simulink model "ardupilotsailboat"  (R2024a)
settings: Solver=ode15s  StartTime=0.0  StopTime=2  RelTol=1e-3
values from neighbouring files (symbols this model uses):
  Ixx = 1/120 * pi * rho * L * B * T * (4*T^2 + B^2)    (= 0.835683076278)    [parameterCalculations.m]
  Izz = 1/120 * pi * rho * L * B * T * (B^2 + L^2)    (= 1.17027496573)    [parameterCalculations.m]
  m = 2.7    [parameterCalculations.m]
  m11 = m*k11    [parameterCalculations.m]
  m22 = m*k22    [parameterCalculations.m]
  m24 = 0    [parameterCalculations.m]
  m26 = xb*m22    [parameterCalculations.m]
  m66 = k66*Izz    [parameterCalculations.m]
  Nr = -pi * T^2/L^2 * (0.25 +0.039 * B/T - 0.56 * B/L)    (= -0.104988463049)    [parameterCalculations.m]
  Nv = -pi * T^2/L^2 * (0.5 +2.4 * T/L)    (= -0.841300100031)    [parameterCalculations.m]
  Yv = -pi * T^2/L^2 * (1 +0.4 * CB * B/T)    (= -0.560439243466)    [parameterCalculations.m]
undefined symbols (not defined in the file or in its folder): Waypoints
libraries: cstblocks x6, simulink x4, vrlib x1
(part 1 of 2)
settings Model: Creator=ruben  LastModifiedBy=ruben
settings SolverCC: MaxConsecutiveZCs=10  MaxConsecutiveMinStep=12  ZeroCrossControl=EnableAll  ZeroCrossAlgorithm=Adaptive  SolverResetMethod=Robust  DecoupledContinuousIntegration=on
settings OptimizationCC: ReuseModelBlockBuffer=off
settings DebuggingCC: SignalInfNanChecking=warning  AlgebraicLoopMsg=error  ArtificialAlgebraicLoopMsg=error  BlockPriorityViolationMsg=error  MinStepSizeMsg=error  MaskedZcDiagnostic=error  IgnoredZcDiagnostic=none  MultiTaskCondExecSysMsg=warning  MultiTaskRateTransMsg=warning  CheckMatrixSingularityMsg=error  StateNameClashWarn=warning
settings RTWCC: GPUComputeCapability=3.5

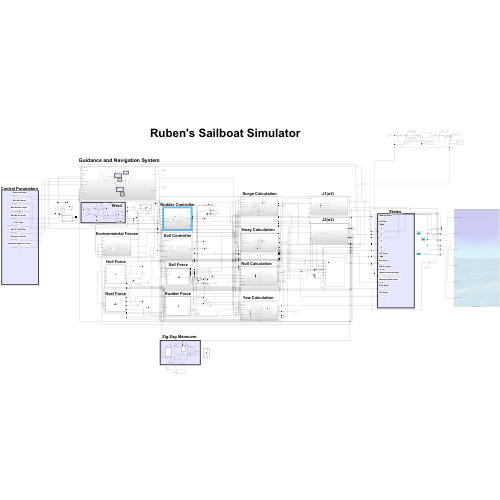
[thumbnail: Simulink's stored preview of the top-level diagram]
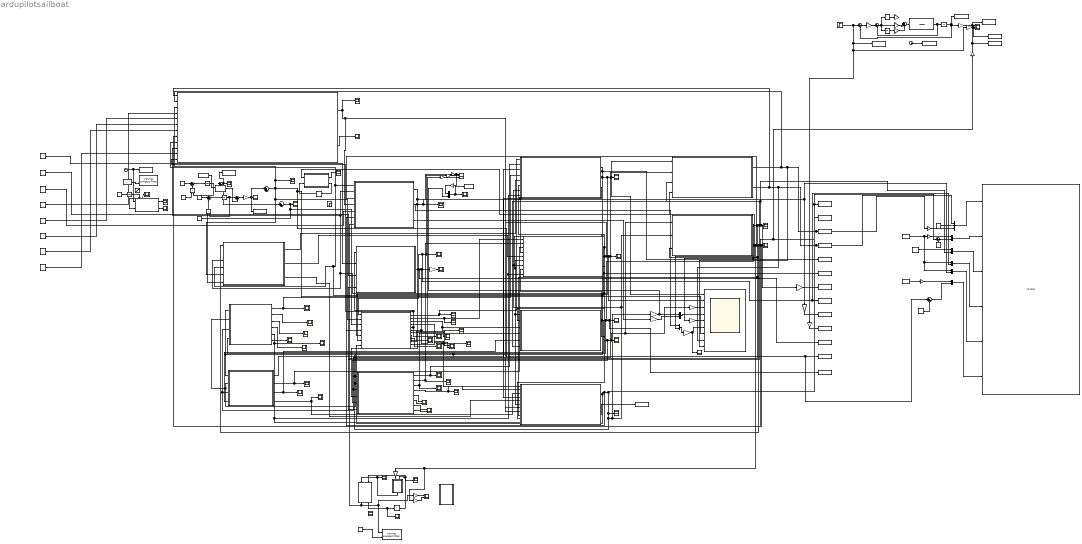
== system ardupilotsailboat ==
  note: Sail Force
  note: Ruben's Sailboat Simulator
  note: States
  note: x
  note: y
  note: Yaw Rate
  note: Heading Angle
  note: u
  note: v
  note: Roll Angle
  note: Sail Angle
  note: Rudder Angle
  note: Desired Heading Angle
  note: Apparent Wind Angle
  note: Wind Angle
  note: Roll Angle
  note: Guidance and Navigation System
  note: Environmental Forces
  note: Surge Calculation
  note: Sway Calculation
  note: Roll Calculation
  note: Yaw Calculation
  note: Wind
  note: Rudder Force
  note: Keel Force
  note: Hull Force
  note: Sail Controller
  note: Rudder Controller
  note: Zig-Zag Maneuver
  note: Control Parameters
  note: Max Sail Angle
  note: Min Sail Angle
  note: Sail No Go Angle
  note: Sail X-Track Max
  note: Waypoint Approach Side
  note: Waypoint Radius
  note: Tack Type
  note: Max Rudder Angle
  note: J1(n2)
  note: J2(n2)
  Band-Limited White Noise : simulink/Sources/Band-Limited White Noise  Cov=[0.05]  Ts=0.25  seed=[23341]
  Band-Limited White Noise1 : simulink/Sources/Band-Limited White Noise  Cov=[0.2]  Ts=0.01  seed=[3341]
  Band-Limited White Noise2 : simulink/Sources/Band-Limited White Noise  Cov=[0.4]  Ts=0.01  seed=[23341]
  Bus Creator : BusCreator  Inputs=2
  Bus Creator1 : BusCreator  Inputs=2
  Bus Creator2 : BusCreator  Inputs=2
  Clock : Clock
  Clock2 : Clock
  Constant : Constant  Value=0.5
  Constant1 : Constant  Value=1.56
  Constant2 : Constant  Value=0.5
  Constant3 : Constant  Value=0
  Cross-Track Distance(m) : Constant  Value=10
  Delay1 : Delay  DelayLength=1  SampleTime=0.01
  Delay2 : Delay  DelayLength=1  SampleTime=0.01
  Derivative : Derivative
  Gain : Gain  Gain=0.0225
  Gain{1..7,12..19,21..22} (17 alike) : Gain  Gain=180/pi
  Gain10 : Gain  Gain=0.332
  Gain11 : Gain
  Gain20 : Gain
  Gain23 : Gain
  Gain8 : Gain  Gain=-180/pi
  Gain9 : Gain  Gain=0.667
  Integrator{,1..2,4} (4 alike) : Integrator
  Integrator3 : Integrator  UpperSaturationLimit=1.3  LowerSaturationLimit=-1.3
  MATLAB Function1 : MATLAB Function  TreatAsAtomicUnit=on
  MATLAB Function2 : MATLAB Function  TreatAsAtomicUnit=on
  MATLAB Function3 : MATLAB Function  TreatAsAtomicUnit=on
  MATLAB Function4 : MATLAB Function  TreatAsAtomicUnit=on
  MATLAB Function5 : MATLAB Function  TreatAsAtomicUnit=on
  MATLAB Function6 : MATLAB Function  TreatAsAtomicUnit=on
  MATLAB Function7 : MATLAB Function  TreatAsAtomicUnit=on
  MATLAB Function8 : MATLAB Function  TreatAsAtomicUnit=on
  MATLAB Function9 : MATLAB Function  TreatAsAtomicUnit=on
  Mux1 : Mux  Inputs=3
  Mux{2,4..7} (5 alike) : Mux  Inputs=2
  "Port: 0, Starboard:1" : Constant  Value=0
  Product : Product
  Product1 : Product
  Radius of Acceptance(m) : Constant  Value=5
  Roll Axis of Rotation : Constant  Value=[ 1 0 0 ]
  Saturation1 : Saturate  UpperLimit=pi/18  LowerLimit=-pi/18
  Scope{,1..14,16..17,19..30,33..35,37..40,42..44} (39 alike) : Scope
  Scope15 : Scope  NumInputPorts=3
  Scope18 : Scope  NumInputPorts=3
  Scope31 : Scope  NumInputPorts=2
  Scope32 : Scope  NumInputPorts=2
  Scope36 : Scope  NumInputPorts=9
  Scope41 : Scope  NumInputPorts=2
  Step : Step  After=0  SampleTime=0
  Step2 : Step  After=0.25  SampleTime=0
  Subsystem1 : Subsystem
  Subsystem10 : Subsystem
  Subsystem2 : Subsystem
  Subsystem3 : Subsystem
  Subsystem4 : Subsystem
  Subsystem5 : Subsystem
  Subsystem6 : Subsystem
  Subsystem7 : Subsystem
  Subsystem8 : Subsystem
  Subsystem9 : Subsystem
  Sum{,5,8,10} (4 alike) : Sum  Inputs=|++
  Sum1 : Sum  Inputs=|+-  SaturateOnIntegerOverflow=on
  Sum{2,4,6..7,9} (5 alike) : Sum  Inputs=|+-
  Sum3 : Sum  Inputs=|+++
  "Tack Type (1:Direct, 2:Indirect 3:Zone)" : Constant
  To File : ToFile  Filename=sim_step.mat  SaveFormat=Timeseries
  To Workspace : ToWorkspace  VariableName=yawrate  SaveFormat=Timeseries  SampleTime=-1
  To Workspace1 : ToWorkspace  VariableName=yaw  SaveFormat=Timeseries  SampleTime=-1
  To Workspace10 : ToWorkspace  VariableName=psid  SaveFormat=Timeseries  SampleTime=-1
  To Workspace11 : ToWorkspace  VariableName=awa  SaveFormat=Timeseries  SampleTime=-1
  To Workspace12 : ToWorkspace  VariableName=wind  SaveFormat=Timeseries  SampleTime=-1
  To Workspace13 : ToWorkspace  VariableName=roll  SaveFormat=Timeseries  SampleTime=-1
  To Workspace14 : ToWorkspace  VariableName=time1  SaveFormat=Timeseries  SampleTime=-1
  To Workspace15 : ToWorkspace  VariableName=time  SaveFormat=Timeseries  SampleTime=-1
  To Workspace16 : ToWorkspace  VariableName=step  SaveFormat=Timeseries  SampleTime=-1
  To Workspace17 : ToWorkspace  VariableName=firstOrder  SaveFormat=Timeseries  SampleTime=-1
  To Workspace18 : ToWorkspace  VariableName=stepInput  SaveFormat=Timeseries  SampleTime=-1
  To Workspace19 : ToWorkspace  VariableName=nonLinear  SaveFormat=Timeseries  SampleTime=-1
  To Workspace2 : ToWorkspace  VariableName=simout  SaveFormat=Timeseries  SampleTime=-1
  To Workspace20 : ToWorkspace  VariableName=yawaccel  SaveFormat=Timeseries  SampleTime=-1
  To Workspace21 : ToWorkspace  VariableName=speed  SaveFormat=Timeseries  SampleTime=-1
  To Workspace22 : ToWorkspace  VariableName=direction  SaveFormat=Timeseries  SampleTime=-1
  To Workspace3 : ToWorkspace  VariableName=x  SaveFormat=Timeseries  SampleTime=-1
  To Workspace4 : ToWorkspace  VariableName=y  SaveFormat=Timeseries  SampleTime=-1
  To Workspace5 : ToWorkspace  VariableName=u  SaveFormat=Timeseries  SampleTime=-1
  To Workspace6 : ToWorkspace  VariableName=v  SaveFormat=Timeseries  SampleTime=-1
  To Workspace7 : ToWorkspace  VariableName=phi  SaveFormat=Timeseries  SampleTime=-1
  To Workspace8 : ToWorkspace  VariableName=delta_s  SaveFormat=Timeseries  SampleTime=-1
  To Workspace9 : ToWorkspace  VariableName=delta_r  SaveFormat=Timeseries  SampleTime=-1
  Transfer Fcn : TransferFcn  Numerator=[2.1]  Denominator=[0.1 1 ]
  VR Sailing Yacht Animation : vrlib/VR Sink  InstantiateOnLoad=on  SampleTime=0.05  ViewEnable=on  RemoteChange=off  RemoteView=off  FieldsWritten=Hull_EarthFixed.translation.3.1.1.double#Rot_Yaw.rotation.4.1.1.double#Rot_Roll.rotation.4.1.1.double#Sail.rotation.4.1.1.double#Rudder.rotation.4.1.1.double#Wind_Arrow.rotation.4.1.1.double  WorldFileName=SailingYachtAnimation.wrl  WorldDescription=Sailing Yacht VR animation  AutoView=on  VideoDimensions=[]  AllowVariableSize=off  FigureProperties="{'Position', 'Name', 'Viewpoint', 'CameraBound', 'CameraDirection', 'CameraPosition', 'CameraUpVector', 'ZoomFactor', 'Antialiasing', 'Headlight', 'Lighting', 'Sound', 'StatusBar', 'Stereo3D', 'Stereo3DCameraOffset', 'Stereo3DHIT', 'ToolBar', 'Textures', 'Transparency', 'Triad', 'Wireframe', 'NavZones', 'NavMode', 'NavSpeed', 'CaptureFileFormat', 'CaptureFileName', 'Record2DCompressMethod', 'Record2DCompressQuality', 'Record2D', 'Record2DFileName', 'Record2DFPS', 'NavPanel'; [-1.9180000000000000e+03   1.6800000000000000e+02   9.5800000000000000e+02   3.8000000000000000e+02], 'Sailing Yacht VR animation', 'Stern', 'on', [4.7333818472333400e-01  -2.7328284422274179e-01  -8.3741713019040154e-01], [-6.4413875659303592e+00   1.1181180118629433e+01   1.9816976942940634e+01], [9.7174256959609767e-02   9.6105616995744136e-01  -2.5870485494298978e-01], [1.0000000000000000e+00], 'on', 'on', 'on', 'on', 'on', 'off', [1.0000000149011612e-01], [0.0000000000000000e+00], 'on', 'on', 'on', 'none', 'off', 'off', 'fly', 'normal', 'tif', '%f_anim_%n.tif', 'auto', [7.5000000000000000e+01], 'off', '%f_anim_%n.avi', 'auto', 'halfbar'}"
  Varying Lowpass Filter : cstblocks/Linear Parameter Varying/Varying Lowpass Filter  N=1
  Varying Lowpass Filter1 : cstblocks/Linear Parameter Varying/Varying Lowpass Filter  N=1
  Yaw Axis of Rotation : Constant  Value=[ 0 1 0 ]
  Yaw Axis of Rotation1 : Constant  Value=[ 0 1 0 ]
  apparent wind : Scope
  fr2 : Constant  Value=20
  freq : Constant  Value=2
  max rudder angle(Rad) : Constant  Value=pi/6
  max sail angle(Rad) : Constant  Value=pi/3
  min sail angle(Rad) : Constant  Value=-pi/3
  pi : Constant  Value=pi
  rudder and psi1 : Scope  NumInputPorts=2
  rudder angle{1,5..6,8} (4 alike) : Scope
  rudder_angle1 : Scope
  rudder_angle2 : Scope
  sail angle : Scope
  sail no go angle(Degrees) : Constant  Value=60
  z : Constant  Value=0
  z - y1 : Gain
  z - y2 : Gain  Gain=-1
  z - y3 : Gain
  z1 : Constant  Value=pi/2
  wires:
  Subsystem1/2(heading (degrees)) -> Scope33/1
  MATLAB Function3/2(Ys) -> Scope1/1, Subsystem4/1(sail force (Ys))
  MATLAB Function3/3(Ks) -> Scope14/1, Subsystem5/3(sail force (Ks))
  MATLAB Function3/4(Ns) -> Subsystem6/1(sail force (Ns)), Scope23/1
  MATLAB Function4/2(Yr) -> Scope2/1, Subsystem4/2(rudder force (Yr))
  MATLAB Function4/3(Kr) -> Scope13/1, Subsystem5/4(roll angle)
  MATLAB Function5/1(Xk) -> Subsystem2/3(keel force (Xk))
  MATLAB Function5/2(Yk) -> Scope3/1, Subsystem4/3(keel force (Yk))
  MATLAB Function5/3(Kk) -> Scope12/1, Subsystem5/5(keel force (Kk))
  MATLAB Function5/4(Nk) -> Scope25/1, Subsystem6/3(keel force (Nk))
  MATLAB Function6/1(Xh) -> Scope5/1, Subsystem2/4(hull force (Xh))
  MATLAB Function6/3(Kh) -> Scope11/1
  MATLAB Function6/4(Nh) -> Scope24/1
  Subsystem4/1(v) -> To Workspace6/1, MATLAB Function3/6(v), Subsystem2/6(v), Subsystem6/7(v), Scope36/2, Scope8/1, Subsystem9/2(v), MATLAB Function6/3(v), MATLAB Function5/3(v), MATLAB Function4/3(v), Subsystem5/2(v), Subsystem8/2(v), Subsystem1/10(v), Subsystem3/3(v)
  Subsystem3/1(Xe) -> Subsystem2/5(environmental force (Xe))
  Subsystem3/2(Ye) -> Subsystem4/5(environmental force (Ye))
  Subsystem3/3(Ne) -> Subsystem6/5(environmental force (Ne))
  Subsystem2/1(u) -> MATLAB Function5/2(u), MATLAB Function6/2(u), MATLAB Function4/2(u), Subsystem1/9(u), Subsystem8/1(u), Subsystem3/4(u), Subsystem6/6(u), Subsystem5/1(u), Subsystem4/6(u), MATLAB Function3/5(u), Scope36/1, Subsystem9/1(u), Scope35/1, To Workspace5/1
  Subsystem5/1(p) -> MATLAB Function4/5(p), Subsystem10/1(p), Gain5/1, Scope38/1, Subsystem4/8(p)
  Subsystem10/1(Phi) -> Gain3/1, MATLAB Function5/4(phi), MATLAB Function6/4(phi), To Workspace13/1, Scope37/1, Subsystem6/9(roll), Subsystem7/4(roll_angle), Subsystem10/3(phi), MATLAB Function4/6(phi), Subsystem9/3(phi), Gain22/1, Scope9/1, Subsystem5/6(rudder force (Kr)), Mux6/2
  Clock2/1 -> MATLAB Function2/1(t), To Workspace14/1
  MATLAB Function7/2(nextState) -> rudder angle5/1, Delay1/1
  Delay1/1 -> rudder angle8/1, MATLAB Function8/2(state), MATLAB Function7/2(currentState)
  MATLAB Function8/1(y) -> MATLAB Function7/1(r), rudder angle1/1
  Gain2/1 -> rudder and psi1/1
  Subsystem7/1(sail angle) -> Gain7/1, sail angle/1, Mux5/2, To Workspace8/1, MATLAB Function3/1(delta_s)
  MATLAB Function3/6(alpha_aw) -> Gain6/1, To Workspace11/1, Gain14/1
  Subsystem8/1(rudder angle) -> Gain8/1, Gain18/1, Mux7/2, rudder_angle1/1, MATLAB Function4/4("delta_r ")
  MATLAB Function4/5(delta_r) -> Scope41/1
  MATLAB Function4/6(alpha_a) -> Scope41/2
  max sail angle(Rad)/1 -> Subsystem7/2(max sail angle)
  min sail angle(Rad)/1 -> Subsystem7/3(min sail angle)
  max rudder angle(Rad)/1 -> Subsystem8/5(max rudder angle)
  sail no go angle(Degrees)/1 -> Subsystem1/4(no go Angle)
  "Tack Type (1:Direct, 2:Indirect 3:Zone)"/1 -> Subsystem1/5(tack Type)
  Cross-Track Distance(m)/1 -> Subsystem1/6(Cross-Track Distance)
  Radius of Acceptance(m)/1 -> Subsystem1/7(radius of acceptance)
  Gain23/1 -> Sum/1, To Workspace22/1, Scope43/1
  MATLAB Function6/5(Frh) -> Scope6/1
  MATLAB Function3/1(Xs) -> Subsystem2/1(sail force (Xs)), Scope7/1
  Subsystem9/2(y) -> Subsystem1/1(x position of Sailboat), Scope36/8, Mux1/1, To Workspace3/1
  Subsystem8/2(Desired Heading) -> Bus Creator/1
  Subsystem10/2(Psi) -> MATLAB Function1/1(psi), Bus Creator/2, Subsystem9/4(psi), Gain17/1, Sum1/1, To Workspace1/1, Subsystem1/8(psi), MATLAB Function3/4(psi), Scope10/1, Subsystem3/1(psi), Subsystem8/3(psi), Gain12/1, Gain13/1
  Bus Creator/1 -> Gain1/1
  z1/1 -> Sum1/2
  z - y1/1 -> Mux4/1
  Yaw Axis of Rotation/1 -> Mux5/1, Mux7/1, z - y1/1
  z/1 -> Mux1/2
  z - y3/1 -> Mux2/1
  Mux2/1 -> VR Sailing Yacht Animation/6
  Sum1/1 -> Mux4/2
  Yaw Axis of Rotation1/1 -> z - y3/1
  z - y2/1 -> Mux1/3
  Roll Axis of Rotation/1 -> Mux6/1
  Mux1/1 -> VR Sailing Yacht Animation/1
  Mux4/1 -> VR Sailing Yacht Animation/2
  Mux6/1 -> VR Sailing Yacht Animation/3
  Mux5/1 -> VR Sailing Yacht Animation/4
  Mux7/1 -> VR Sailing Yacht Animation/5
  Subsystem9/1(x) -> Subsystem1/2(y position of Sailboat), Scope36/9, z - y2/1, To Workspace4/1
  MATLAB Function3/5(awa) -> Subsystem7/1(apparent_wind_angle), Subsystem1/12(awa), Scope42/1
  Gain3/1 -> Scope36/5
  Gain1/1 -> Scope19/1, Scope36/6
  Gain4/1 -> Bus Creator2/1, Bus Creator1/2
  Gain5/1 -> Scope36/3
  Gain6/1 -> Scope15/3
  Gain7/1 -> Scope15/2
  Gain8/1 -> Gain20/1, Scope15/1
  MATLAB Function1/2(nextState) -> Delay2/1
  Delay2/1 -> MATLAB Function1/2(currentState)
  MATLAB Function1/1(y) -> Scope16/1
  Clock/1 -> To Workspace15/1
  Integrator/1 -> Gain10/1
  Derivative/1 -> Gain/1
  Gain9/1 -> Sum3/2
  Transfer Fcn/1 -> Sum2/2, Integrator1/1
  Sum2/1 -> Derivative/1, Gain9/1, Integrator/1
  Sum3/1 -> Transfer Fcn/1
  Gain10/1 -> Sum3/3
  Step2/1 -> Sum4/1, Gain21/1, Gain16/1, To Workspace16/1
  Integrator1/1 -> Sum4/2, Gain15/1, To Workspace2/1
  Sum4/1 -> Gain11/1
  Gain11/1 -> Sum2/1
  Subsystem1/1(heading (rad)) -> Scope/1, Subsystem8/4(desired heading), Subsystem6/8(desired heading)
  "Port: 0, Starboard:1"/1 -> Subsystem1/11(waypoint approach)
  Subsystem6/1(r) -> Subsystem8/6(r), MATLAB Function5/1(r), MATLAB Function6/1(r), MATLAB Function4/1(r), Gain4/1, Subsystem10/2(r), Subsystem2/7(r), Subsystem4/7(r), Scope40/1, To Workspace/1, MATLAB Function3/7(r)
  Gain12/1 -> rudder and psi1/2
  Gain13/1 -> MATLAB Function8/1(psi)
  fr2/1 -> Varying Lowpass Filter/2
  MATLAB Function7/1(y) -> Gain2/1, Varying Lowpass Filter/1, Subsystem8/7(zig zag)
  Gain14/1 -> apparent wind/1
  Gain15/1 -> To Workspace17/1, Scope18/1
  Gain16/1 -> To Workspace18/1, Scope18/2
  Gain17/1 -> Scope18/3, To Workspace19/1
  Gain18/1 -> To Workspace9/1
  Bus Creator1/1 -> To File/1, rudder_angle2/1
  MATLAB Function4/4(Nr) -> Scope21/1, Subsystem6/2(rudder force (Nr))
  Gain20/1 -> Bus Creator1/1
  MATLAB Function4/1(Xr) -> Subsystem2/2(rudder force (Xr)), Scope22/1
  Bus Creator2/1 -> Scope36/4
  Gain19/1 -> Bus Creator2/2
  Subsystem8/3(desired yaw rate) -> Gain19/1
  Subsystem6/2(rdot) -> To Workspace20/1
  Sum/1 -> Subsystem1/3(wind angle), Scope17/1, Scope36/7, Sum6/1, To Workspace12/1, MATLAB Function3/2(wind_direction), Subsystem3/5(wind Direction)
  MATLAB Function3/7(apparent_velocity) -> Scope20/1
  MATLAB Function3/8(V_awu) -> Scope26/1
  MATLAB Function3/9(V_awv) -> Scope27/1
  Sum5/1 -> Scope34/1, Subsystem3/6(wind Velocity), MATLAB Function3/3(wind_velocity)
  freq/1 -> Varying Lowpass Filter1/2
  Band-Limited White Noise/1 -> Integrator3/1
  MATLAB Function2/2(direction) -> Scope29/1
  MATLAB Function4/7(lift_force) -> Scope31/1
  MATLAB Function4/8(drag_force) -> Scope31/2
  Subsystem4/2(v dot) -> Subsystem6/10(vdot)
  ? -> Sum5/2
  MATLAB Function2/1(amplitude) -> Scope30/1
  MATLAB Function3/10(L) -> Scope32/1
  MATLAB Function3/11(D) -> Scope32/2
  Sum6/1 -> Mux2/2
  pi/1 -> Sum6/2
  Integrator3/1 -> Scope28/1, MATLAB Function2/2(gust_direction)
  Gain21/1 -> To Workspace10/1
  ? -> ?
  MATLAB Function6/2(Yh) -> Scope4/1
  Sum8/1 -> Sum5/1, To Workspace21/1, Scope39/1
  Gain22/1 -> To Workspace7/1
  Constant/1 -> Product/1
  Product/1 -> Sum7/2
  Constant1/1 -> Sum8/2
  Integrator4/1 -> Product/2
  Sum7/1 -> Integrator4/1
  Band-Limited White Noise2/1 -> Sum7/1
  Band-Limited White Noise1/1 -> Sum9/1
  Constant3/1 -> Sum10/2
  Product1/1 -> Sum9/2
  Integrator2/1 -> Sum10/1, Product1/2
  Constant2/1 -> Product1/1
  Sum10/1 -> Gain23/1
  Sum9/1 -> Integrator2/1
  MATLAB Function6/6(alpha_ah) -> Subsystem6/11(hull_ah), Subsystem2/8(hull_ah), Subsystem4/9(hull_ah), Scope44/1
  Subsystem2/2(hull) -> Subsystem6/4(hull force (Nh)), Subsystem4/4("hull force ")

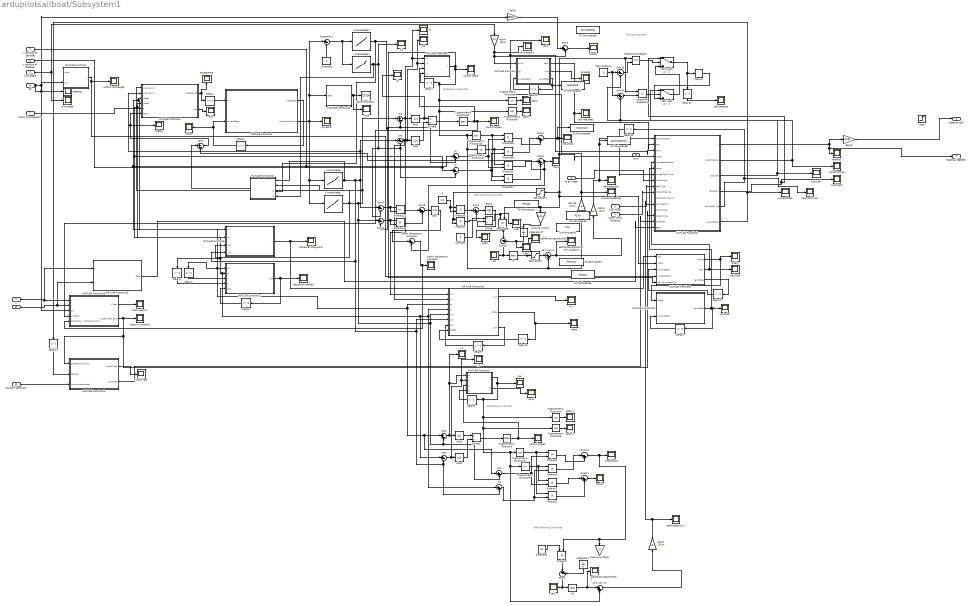
== system ardupilotsailboat/Subsystem1 ==
  note: Guidance Axis System
  note: Tacking Controller
  note: Path Following Controller
  note: Guidance Axis System
  note: Path Following Controller
  x position of Sailboat : Inport
  y position of Sailboat : Inport  Port=2
  wind angle : Inport  Port=3
  no go Angle : Inport  Port=4
  tack Type : Inport  Port=5
  Cross-Track Distance : Inport  Port=6
  radius of acceptance : Inport  Port=7
  psi : Inport  Port=8
  u : Inport  Port=9
  v : Inport  Port=10
  waypoint approach : Inport  Port=11
  awa : Inport  Port=12
  " heading" : Scope
  " wind angle" : Scope
  Abs{1..4} (4 alike) : Abs  SaturateOnIntegerOverflow=off
  Constant : Constant
  Constant1 : Constant  Value=0.2
  Constant2 : Constant
  Delay{1..2,4..12,14..15} (13 alike) : Delay  DelayLength=1
  Delay13 : Delay  DelayLength=1  SampleTime=2
  Delay3 : Delay  DelayLength=1  SampleTime=2
  Divide : Product  Inputs=*/
  Divide1 : Product  Inputs=*/
  Divide6 : Product  Inputs=*/
  Gain{1..2,4..5,15} (5 alike) : Gain  Gain=180/pi
  Gain3 : Gain  Gain=pi/180
  Integrator1 : Integrator  LimitOutput=on  UpperSaturationLimit=10  LowerSaturationLimit=-10
  Integrator17 : Integrator  LimitOutput=on  UpperSaturationLimit=pi/10  LowerSaturationLimit=-pi/10
  Kpe : Scope
  Kpe1 : Scope
  Kpe2 : Scope
  MATLAB Function1 : MATLAB Function  TreatAsAtomicUnit=on
  MATLAB Function10 : MATLAB Function  TreatAsAtomicUnit=on
  MATLAB Function11 : MATLAB Function  TreatAsAtomicUnit=on
  MATLAB Function12 : MATLAB Function  TreatAsAtomicUnit=on
  MATLAB Function13 : MATLAB Function  TreatAsAtomicUnit=on
  MATLAB Function14 : MATLAB Function  TreatAsAtomicUnit=on
  MATLAB Function15 : MATLAB Function  TreatAsAtomicUnit=on
  MATLAB Function16 : MATLAB Function  TreatAsAtomicUnit=on
  MATLAB Function18 : MATLAB Function  TreatAsAtomicUnit=on
  MATLAB Function2 : MATLAB Function  TreatAsAtomicUnit=on
  MATLAB Function3 : MATLAB Function  TreatAsAtomicUnit=on
  MATLAB Function4 : MATLAB Function  TreatAsAtomicUnit=on
  MATLAB Function5 : MATLAB Function  TreatAsAtomicUnit=on
  MATLAB Function6 : MATLAB Function  TreatAsAtomicUnit=on
  MATLAB Function7 : MATLAB Function  TreatAsAtomicUnit=on
  MATLAB Function8 : MATLAB Function  TreatAsAtomicUnit=on
  MATLAB Function9 : MATLAB Function  TreatAsAtomicUnit=on
  Memory : Memory
  Product{1..7,10..13,84..85,88} (14 alike) : Product
  R : Constant  Value=4.1
  Relational Operator : RelationalOperator  Operator=<=  OutDataTypeStr=boolean  RndMeth=Simplest  InputSameDT=off
  Relational Operator1 : RelationalOperator  Operator=>  OutDataTypeStr=boolean  RndMeth=Simplest  InputSameDT=off
  Saturation1 : Saturate  UpperLimit=4  LowerLimit=-4
  Saturation2 : Saturate  UpperLimit=pi/2  LowerLimit=-pi/2
  Scope1 : Scope
  Scope33 : Scope
  Sqrt : Sqrt
  Sqrt1 : Sqrt
  Step : Step  After=0.25  SampleTime=0
  Stop Simulation : Stop
  Sum1 : Sum  Inputs=|--
  Sum{2..3,9..11} (5 alike) : Sum  Inputs=|+-
  Sum14 : Sum  Inputs=|++
  Sum16 : Sum  Inputs=|--
  Sum8 : Sum  Inputs=|++
  Tack Direction : Constant  Value=0
  Tack Left : Switch  Criteria=u2 > Threshold  SaturateOnIntegerOverflow=off  InputSameDT=off
  Tack Right : Switch  Criteria=u2 > Threshold  SaturateOnIntegerOverflow=off  InputSameDT=off
  To Workspace1 : ToWorkspace  VariableName=PCKi  SaveFormat=Timeseries  SampleTime=-1
      settings: Decimation=4
  To Workspace2 : ToWorkspace  VariableName=PCKpG  SaveFormat=Timeseries  SampleTime=-1
      settings: Decimation=4
  To Workspace3 : ToWorkspace  VariableName=PCKp  SaveFormat=Timeseries  SampleTime=-1
      settings: Decimation=4
  To Workspace4 : ToWorkspace  VariableName=PCTotal  SaveFormat=Timeseries  SampleTime=-1
      settings: Decimation=4
  To Workspace5 : ToWorkspace  VariableName=PCatan  SaveFormat=Timeseries  SampleTime=-1
      settings: Decimation=4
  To Workspace6 : ToWorkspace  VariableName=crosstrack  SaveFormat=Timeseries  SampleTime=-1
  To Workspace7 : ToWorkspace  VariableName=tackState  SaveFormat=Timeseries  SampleTime=-1
  To Workspace8 : ToWorkspace  VariableName=pathtrajectory  SaveFormat=Timeseries  SampleTime=-1
  To Workspace9 : ToWorkspace  VariableName=tackheading  SaveFormat=Timeseries  SampleTime=-1
  Trigonometric Function1 : Trigonometry  Operator=atan
  Trigonometric Function15 : Trigonometry  Operator=atan
  Trigonometric Function{2,5,9,16} (4 alike) : Trigonometry  Operator=cos
  Trigonometric Function{3..4,8,17} (4 alike) : Trigonometry
  Waypoint-1 : Sum  Inputs=|+-
  acceptance : Scope
  angle : Scope
  causing windup : Gain  Gain=0.01
  causing windup1 : Gain  Gain=0
  close to waypoint : Scope
  control angle : Scope
  control angle1 : Scope
  control angle2 : Scope
  control wind angle : Scope
  crosstrack : Scope
  crosstrack1 : Scope
  currentState : Scope
  dist : Scope
  distance travelled : Scope
  distanceToWaypoint : Scope
  heading : Scope
  nextTackType : Scope
  p_w : Scope
  "pathFollowingController+waypoint " : Scope
  pathfollowingcontroller : Scope
  pathfollowingcontroller1 : Scope
  pathtrajectory : Scope
  pathtrajectory1 : Scope
  pathx : Scope
  pathx1 : Scope
  pathy : Scope
  pathy1 : Scope
  psi1 : Scope
  pwu1 : Scope
  state : Scope
  state1 : Scope
  stop : Scope
  switch tack : Scope
  tack required : Scope
  tackDistance : Scope
  tackHeading : Scope
  tackLeft : Scope
  tackRight : Scope
  tackSide : Scope
  tackside : Scope
  tan : Scope
  tan1 : Scope
  theta : Scope
  track : Scope
  track velocity : Scope
  track1 : Scope
  trackx distance to waypoint : Scope
  wayPointHeading : Scope
  waypoint : Scope
  wind angle 3 : Scope
  x-coordinates : Lookup_n-D  NumberOfTableDimensions=1  BreakpointsForDimension1=Waypoints.number  Table=Waypoints.x  InterpMethod=Cubic spline  ExtrapMethod=Cubic spline  InternalRulePriority=Speed  RndMeth=Simplest
  x-coordinates1 : Lookup_n-D  NumberOfTableDimensions=1  BreakpointsForDimension1=Waypoints.number  Table=Waypoints.x  InterpMethod=Cubic spline  ExtrapMethod=Cubic spline  InternalRulePriority=Speed  RndMeth=Simplest
  x{1..4} (4 alike) : Scope
  xd = xp+xr : Sum  Inputs=|++
  xd = xp+xr1 : Sum  Inputs=|++
  xh : Sum  Inputs=|+-
  xh1 : Sum  Inputs=|+-
  xr : Trigonometry  Operator=atan
  xr1 : Trigonometry  Operator=atan
  xsd : Sum  Inputs=|+-
  xsd1 : Sum  Inputs=|+-
  xsd2 : Sum  Inputs=|+-
  xtrack : Sum  Inputs=|++
  xtrack distance to waypoint : Sum  Inputs=|+-
  xtrack1 : Sum  Inputs=|++
  y-coordinates : Lookup_n-D  NumberOfTableDimensions=1  BreakpointsForDimension1=Waypoints.number  Table=Waypoints.y  InterpMethod=Cubic spline  ExtrapMethod=Cubic spline  InternalRulePriority=Speed  RndMeth=Simplest
  y-coordinates1 : Lookup_n-D  NumberOfTableDimensions=1  BreakpointsForDimension1=Waypoints.number  Table=Waypoints.y  InterpMethod=Cubic spline  ExtrapMethod=Cubic spline  InternalRulePriority=Speed  RndMeth=Simplest
  y11 : Scope
  y3 : Scope
  yh : Sum  Inputs=|+-
  yh1 : Sum  Inputs=|+-
  ypw : Scope
  ysd : Sum  Inputs=|+-
  ysd1 : Sum  Inputs=|+-
  ytrack : Sum  Inputs=|-+
  ytrack1 : Sum  Inputs=|-+
  heading (rad) : Outport
  heading (degrees) : Outport  Port=2
  wires:
  MATLAB Function11/2(theta) -> Delay10/1, theta/1
  Delay2/1 -> MATLAB Function4/2(currentState), state/1
  Trigonometric Function17/1 -> Product10/1, Product85/1
  MATLAB Function3/6(currentState) -> Delay14/1, currentState/1
  MATLAB Function3/1(y) -> Gain3/1, heading (degrees)/1, heading/1
  Gain2/1 -> To Workspace8/1, MATLAB Function3/1(pathTrajectory), pathtrajectory/1
  Delay12/1 -> MATLAB Function3/7(currentTackType)
  MATLAB Function4/2(currentWaypoint) -> MATLAB Function10/1(state), Waypoint-1/1, waypoint/1, x-coordinates/1, y-coordinates/1
  yh/1 -> Product85/2, Product11/2
  Sum14/1 -> Relational Operator1/2
  ytrack/1 -> To Workspace6/1, Saturation1/1, Product88/2, causing windup/1, MATLAB Function9/2(xtrack), MATLAB Function3/4(xtrack), crosstrack/1, Relational Operator1/1, Relational Operator/1
  Product85/1 -> ytrack/1
  Delay11/1 -> tackHeading/1
  MATLAB Function3/2(tackDistance) -> Sum10/2, Sum14/2, tackDistance/1
  Integrator17/1 -> Kpe2/1, Sum16/2
  Abs1/1 -> x3/1, Divide6/1
  Trigonometric Function16/1 -> Product11/1, Product84/1
  Delay7/1 -> MATLAB Function8/4(us)
  MATLAB Function18/1(nextState) -> tackside/1, Delay3/1, MATLAB Function3/6(zone)
  xd = xp+xr/1 -> "pathFollowingController+waypoint "/1, Gain2/1
  Gain15/1 -> MATLAB Function3/3(AWA), psi1/1, MATLAB Function7/2(psi), wayPointHeading/1
  MATLAB Function3/5(nextTackType) -> Delay12/1, nextTackType/1
  Delay13/1 -> MATLAB Function9/3(currentState)
  Waypoint-1/1 -> x-coordinates1/1, y-coordinates1/1
  Delay3/1 -> MATLAB Function18/2(currentState)
  xsd/1 -> MATLAB Function11/1(xw), MATLAB Function8/1(x1), x1/1, Abs1/1
  Constant2/1 -> Waypoint-1/2
  MATLAB Function8/1(y) -> Trigonometric Function8/1, Trigonometric Function9/1, Trigonometric Function17/1, xd = xp+xr/2, Gain15/1, Trigonometric Function16/1, Delay7/1, control angle/1, MATLAB Function9/5(wayPointHeading)
  xh/1 -> Product84/2, Product10/2
  Delay1/1 -> MATLAB Function4/1(R)
  MATLAB Function9/3(nextState) -> Delay13/1
  Product84/1 -> ytrack/2
  y-coordinates1/1 -> MATLAB Function16/4(y1), yh/2, ysd/2, Sum9/2, x2/1
  Trigonometric Function15/1 -> MATLAB Function13/4(psiTrack), control angle1/1, MATLAB Function8/3(u)
  ysd/1 -> y11/1, MATLAB Function8/2(y1), Abs2/1, MATLAB Function11/2(yw)
  x-coordinates1/1 -> MATLAB Function16/3(x1), Sum11/2, xh/2, xsd/2
  Sum16/1 -> xr/1, tan/1
  Product13/1 -> Sum8/2
  MATLAB Function6/1(y) -> MATLAB Function9/1(dist), distanceToWaypoint/1
  Delay5/1 -> MATLAB Function12/4(y)
  MATLAB Function9/1(angle) -> angle/1, MATLAB Function18/1(angle)
  Product88/1 -> Sum16/1, Kpe1/1
  Relational Operator1/1 -> Tack Left/2
  MATLAB Function3/3(tackLeft) -> Tack Left/1, tackLeft/1
  Tack Right/1 -> Memory/1, Delay11/1
  xtrack distance to waypoint/1 -> MATLAB Function13/5(trackDistanceToWaypoint), trackx distance to waypoint/1
  Memory/1 -> Tack Left/3
  Product11/1 -> xtrack/2
  Trigonometric Function8/1 -> pathy/1
  MATLAB Function7/1(tack) -> MATLAB Function3/2(tack), tack required/1
  Delay4/1 -> MATLAB Function12/3(x)
  causing windup/1 -> Integrator17/1
  Tack Left/1 -> Tack Right/3
  MATLAB Function10/1(y) -> stop/1, Stop Simulation/1
  Sum8/1 -> Sqrt/1
  Sum11/1 -> Product13/2, Product13/1
  Tack Direction/1 -> Sum14/1, Sum10/1
  Sum9/1 -> Product12/1, Product12/2
  Delay6/1 -> MATLAB Function12/5("dist ")
  MATLAB Function5/1(acceptance) -> Delay1/1, acceptance/1
  MATLAB Function12/1(dist) -> distance travelled/1, Delay6/1
  Relational Operator/1 -> Tack Right/2
  Sum10/1 -> Relational Operator/2
  xtrack/1 -> xsd2/2, xtrack distance to waypoint/2, track/1
  Abs2/1 -> Divide6/2
  MATLAB Function4/1(nextState) -> Delay2/1
  Sqrt/1 -> xtrack distance to waypoint/1
  MATLAB Function11/1(p_w) -> p_w/1
  Product10/1 -> xtrack/1
  xr/1 -> pathfollowingcontroller/1, Saturation2/1
  MATLAB Function3/4(tackRight) -> tackRight/1, Tack Right/1
  Product12/1 -> Sum8/1
  Trigonometric Function9/1 -> pathx/1
  MATLAB Function7/2(awa) -> Scope33/1
  no go Angle/1 -> MATLAB Function3/8(noGoAngle)
  tack Type/1 -> MATLAB Function3/9(tackType)
  Cross-Track Distance/1 -> MATLAB Function3/10(XtrackDistance)
  radius of acceptance/1 -> MATLAB Function5/5(R)
  MATLAB Function9/2(tack) -> MATLAB Function3/5(indirectTackSide), tackSide/1
  MATLAB Function5/2(dist) -> dist/1
  wind angle/1 -> " wind angle"/1, Gain4/1
  MATLAB Function1/1(y) -> MATLAB Function9/4(windDirection), control wind angle/1
  Divide6/1 -> Trigonometric Function15/1
  Divide1/1 -> Trigonometric Function1/1
  Product2/1 -> xtrack1/2
  Trigonometric Function5/1 -> pathx1/1
  Product1/1 -> xtrack1/1
  Abs4/1 -> Divide1/2
  Trigonometric Function4/1 -> pathy1/1
  y-coordinates/1 -> MATLAB Function16/1(x), yh1/2, ysd1/2, MATLAB Function11/6(ycw), MATLAB Function6/4(ywp), MATLAB Function5/2(yWaypoint), ysd/1, Sum9/1
  xtrack1/1 -> track1/1
  xh1/1 -> Product3/2, Product1/2
  Abs3/1 -> Divide1/1
  ysd1/1 -> y3/1, MATLAB Function2/2(y1), Abs4/1
  x-coordinates/1 -> MATLAB Function6/3(xwp), MATLAB Function16/2("y "), xh1/2, xsd1/2, MATLAB Function11/5(xcw), Sum11/1, xsd/1, MATLAB Function5/1(xWaypoint)
  Product3/1 -> ytrack1/2
  Trigonometric Function2/1 -> Product2/1, Product3/1
  Product4/1 -> ytrack1/1
  Trigonometric Function3/1 -> Product1/1, Product4/1
  yh1/1 -> Product4/2, Product2/2
  xsd1/1 -> x4/1, MATLAB Function2/1(x1), Abs3/1
  Trigonometric Function1/1 -> MATLAB Function2/3(u), control angle2/1
  Delay8/1 -> MATLAB Function2/4(us)
  xr1/1 -> xd = xp+xr1/1, pathfollowingcontroller1/1
  Product5/1 -> Sum1/1
  Constant1/1 -> Product5/1
  Sum1/1 -> xr1/1, tan1/1
  MATLAB Function2/1(y) -> ypw/1, Trigonometric Function4/1, Trigonometric Function5/1, xd = xp+xr1/2, Trigonometric Function3/1, Trigonometric Function2/1, Delay8/1
  xd = xp+xr1/1 -> Gain1/1
  Integrator1/1 -> Sum1/2
  ytrack1/1 -> Product5/2, causing windup1/1, crosstrack1/1
  Gain1/1 -> MATLAB Function3/12(pwTrajectory), pathtrajectory1/1
  MATLAB Function2/2(u1) -> pwu1/1
  x position of Sailboat/1 -> xh/1, xh1/1, xsd1/1, MATLAB Function11/3(xs), MATLAB Function12/1(xs), Delay4/1, MATLAB Function6/1(xw), MATLAB Function5/3(xBoat)
  y position of Sailboat/1 -> yh/1, MATLAB Function6/2(yw), MATLAB Function5/4(yBoat), ysd1/1, yh1/1, MATLAB Function11/4(ys), MATLAB Function12/2(ys), Delay5/1
  MATLAB Function11/3(pwn) -> Delay9/1
  Delay9/1 -> MATLAB Function11/7(pwc)
  Delay10/1 -> MATLAB Function11/8(thetaP)
  Sum2/1 -> Sqrt1/1
  Product6/1 -> Sum2/1
  Product7/1 -> Sum2/2
  Constant/1 -> Divide/1
  Sqrt1/1 -> Divide/2
  Divide/1 -> Product88/1, Kpe/1
  Saturation1/1 -> Product7/2, Product7/1
  v/1 -> MATLAB Function15/2(v), MATLAB Function13/2(v)
  MATLAB Function13/1(uTrack) -> track velocity/1
  MATLAB Function13/2(closeToWaypoint) -> MATLAB Function3/14(closeToWay), MATLAB Function14/1(closeToWaypoint), close to waypoint/1
  MATLAB Function14/1(switchTack) -> switch tack/1
  waypoint approach/1 -> MATLAB Function14/3(waypointApproach)
  Delay14/1 -> MATLAB Function14/2(tacking)
  MATLAB Function14/2(psiOffset) -> MATLAB Function3/15(psiOffset)
  Gain3/1 -> heading (rad)/1
  psi/1 -> Gain5/1, " heading"/1, MATLAB Function1/2(psi), MATLAB Function13/3(psi)
  R/1 -> Product6/2, Product6/1
  Saturation2/1 -> xd = xp+xr/1
  Gain4/1 -> Sum3/2, MATLAB Function7/1(wind), wind angle 3/1
  MATLAB Function7/3(nextState) -> To Workspace7/1, Delay15/1
  Delay15/1 -> MATLAB Function7/3(currentState)
  MATLAB Function15/1(Beta) -> MATLAB Function3/16(Beta)
  u/1 -> MATLAB Function15/1(u), MATLAB Function13/1(u)
  Gain5/1 -> Sum3/1
  Sum3/1 -> Scope1/1
  xsd2/1 -> MATLAB Function5/6(ltrack), state1/1
  MATLAB Function16/1(y) -> xsd2/1

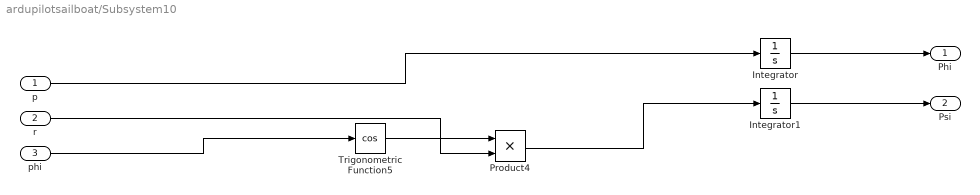
== system ardupilotsailboat/Subsystem10 ==
  p : Inport
  r : Inport  Port=2
  phi : Inport  Port=3
  Integrator : Integrator
  Integrator1 : Integrator
  Product4 : Product
  Trigonometric Function5 : Trigonometry  Operator=cos
  Phi : Outport
  Psi : Outport  Port=2
  wires:
  Integrator1/1 -> Psi/1
  Integrator/1 -> Phi/1
  p/1 -> Integrator/1
  Trigonometric Function5/1 -> Product4/1
  Product4/1 -> Integrator1/1
  r/1 -> Product4/2
  phi/1 -> Trigonometric Function5/1

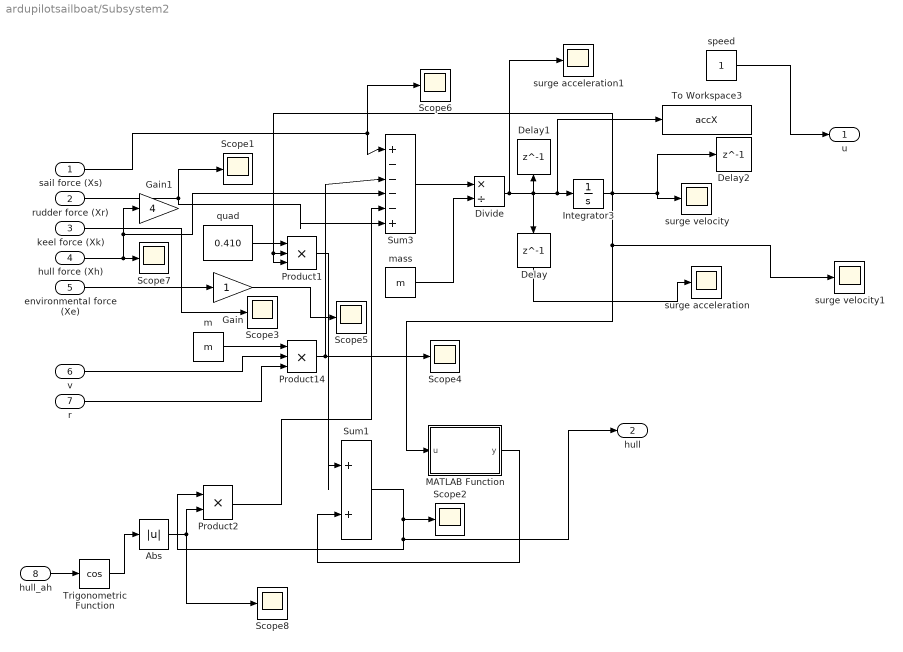
== system ardupilotsailboat/Subsystem2 ==
  sail force (Xs) : Inport
  rudder force (Xr) : Inport  Port=2
  keel force (Xk) : Inport  Port=3
  hull force (Xh) : Inport  Port=4
  environmental force (Xe) : Inport  Port=5
  v : Inport  Port=6
  r : Inport  Port=7
  hull_ah : Inport  Port=8
  Abs : Abs  SaturateOnIntegerOverflow=off
  Delay : Delay  DelayLength=1  InitialCondition=0
  Delay1 : Delay  DelayLength=1  InitialCondition=0
  Delay2 : Delay  DelayLength=1  InitialCondition=0
  Divide : Product  Inputs=*/
  Gain : Gain
  Gain1 : Gain  Gain=4
  Integrator3 : Integrator  InitialCondition=1  LimitOutput=on  UpperSaturationLimit=1.5  LowerSaturationLimit=0
  MATLAB Function : MATLAB Function  TreatAsAtomicUnit=on
  Product1 : Product  Inputs=3
  Product14 : Product  Inputs=3
  Product2 : Product
  Scope{1..8} (8 alike) : Scope
  Sum1 : Sum  Inputs=|++
  Sum3 : Sum  Inputs=|+----+
  To Workspace3 : ToWorkspace  VariableName=accX  SaveFormat=Timeseries  SampleTime=-1
  Trigonometric Function : Trigonometry  Operator=cos
  m : Constant  Value=m
  mass : Constant  Value=m
  quad : Constant  Value=0.410
  speed : Constant
  surge acceleration : Scope
  surge acceleration1 : Scope
  surge velocity : Scope
  surge velocity1 : Scope
  u : Outport
  hull : Outport  Port=2
  wires:
  m/1 -> Product14/1
  mass/1 -> Divide/2
  Sum3/1 -> Divide/1
  rudder force (Xr)/1 -> Sum3/6, Scope1/1
  keel force (Xk)/1 -> Scope3/1
  environmental force (Xe)/1 -> Gain/1
  r/1 -> Product14/3
  v/1 -> Product14/2
  Delay/1 -> surge acceleration/1
  Divide/1 -> Delay/1, Delay1/1, To Workspace3/1, Integrator3/1, surge acceleration1/1
  quad/1 -> Product1/1
  hull force (Xh)/1 -> Sum3/4, Gain1/1, Scope7/1
  Product14/1 -> Sum3/3, Scope4/1
  Integrator3/1 -> Product1/3, Product1/2, MATLAB Function/1(u), surge velocity1/1, Delay2/1, surge velocity/1
  Gain/1 -> Scope5/1
  Product1/1 -> Sum1/1
  sail force (Xs)/1 -> Scope6/1, Sum3/1
  MATLAB Function/1(y) -> Sum1/2
  hull_ah/1 -> Trigonometric Function/1
  Trigonometric Function/1 -> Abs/1
  Sum1/1 -> hull/1, Product2/1, Scope2/1
  Product2/1 -> Sum3/5
  Abs/1 -> Scope8/1, Product2/2
  speed/1 -> u/1

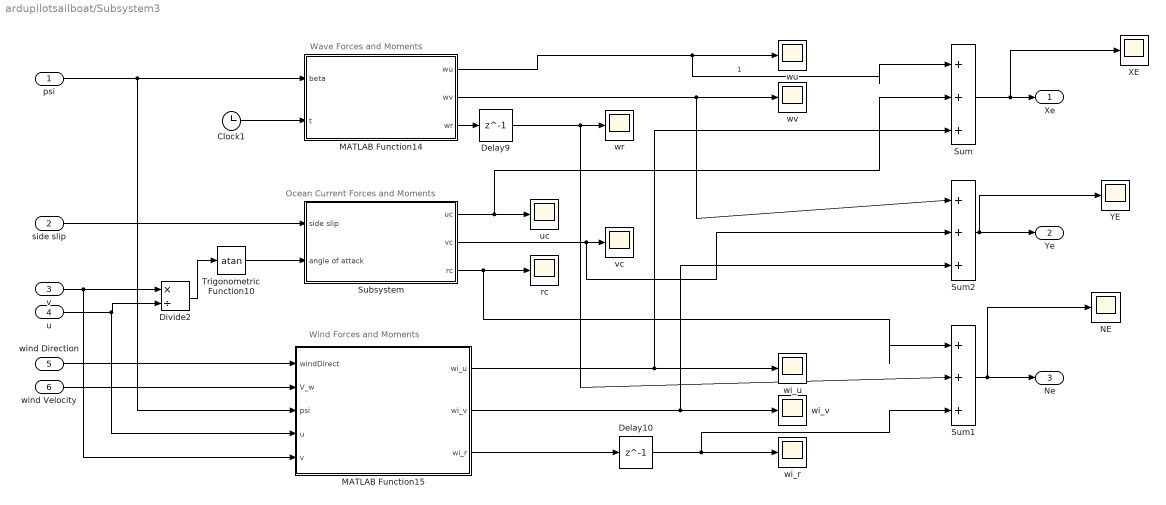
== system ardupilotsailboat/Subsystem3 ==
  note: Wave Forces and Moments
  note: Wind Forces and Moments
  note: Ocean Current Forces and Moments
  psi : Inport
  side slip : Inport  Port=2
  v : Inport  Port=3
  u : Inport  Port=4
  wind Direction : Inport  Port=5
  wind Velocity : Inport  Port=6
  Clock1 : Clock
  Delay10 : Delay  DelayLength=1
  Delay9 : Delay  DelayLength=1
  Divide2 : Product  Inputs=*/
  MATLAB Function14 : MATLAB Function  TreatAsAtomicUnit=on
  MATLAB Function15 : MATLAB Function  TreatAsAtomicUnit=on
  NE : Scope
  Subsystem : Subsystem
  Sum : Sum  Inputs=|+++
  Sum1 : Sum  Inputs=|+++
  Sum2 : Sum  Inputs=|+++
  Trigonometric Function10 : Trigonometry  Operator=atan
  XE : Scope
  YE : Scope
  rc : Scope
  uc : Scope
  vc : Scope
  wi_r : Scope
  wi_u : Scope
  wi_v : Scope
  wr : Scope
  wu : Scope
  wv : Scope
  Xe : Outport
  Ye : Outport  Port=2
  Ne : Outport  Port=3
  wires:
  MATLAB Function14/2(wv) -> Sum2/1, wv/1
  Trigonometric Function10/1 -> Subsystem/2(angle of attack)
  MATLAB Function14/3(wr) -> Delay9/1
  MATLAB Function15/2(wi_v) -> Sum2/3, wi_v/1
  Subsystem/1(uc) -> Sum/2, uc/1
  MATLAB Function15/3(wi_r) -> Delay10/1
  MATLAB Function15/1(wi_u) -> Sum/3, wi_u/1
  Clock1/1 -> MATLAB Function14/2(t)
  Subsystem/2(vc) -> Sum2/2, vc/1
  MATLAB Function14/1(wu) -> Sum/1, wu/1  "1"
  Divide2/1 -> Trigonometric Function10/1
  psi/1 -> MATLAB Function14/1(beta), MATLAB Function15/3(psi)
  side slip/1 -> Subsystem/1(side slip)
  v/1 -> MATLAB Function15/5(v), Divide2/1
  u/1 -> MATLAB Function15/4(u), Divide2/2
  wind Direction/1 -> MATLAB Function15/1(windDirect)
  wind Velocity/1 -> MATLAB Function15/2(V_w)
  Delay10/1 -> Sum1/3, wi_r/1
  Subsystem/3(rc) -> Sum1/1, rc/1
  Delay9/1 -> Sum1/2, wr/1
  Sum/1 -> XE/1, Xe/1
  Sum1/1 -> NE/1, Ne/1
  Sum2/1 -> YE/1, Ye/1

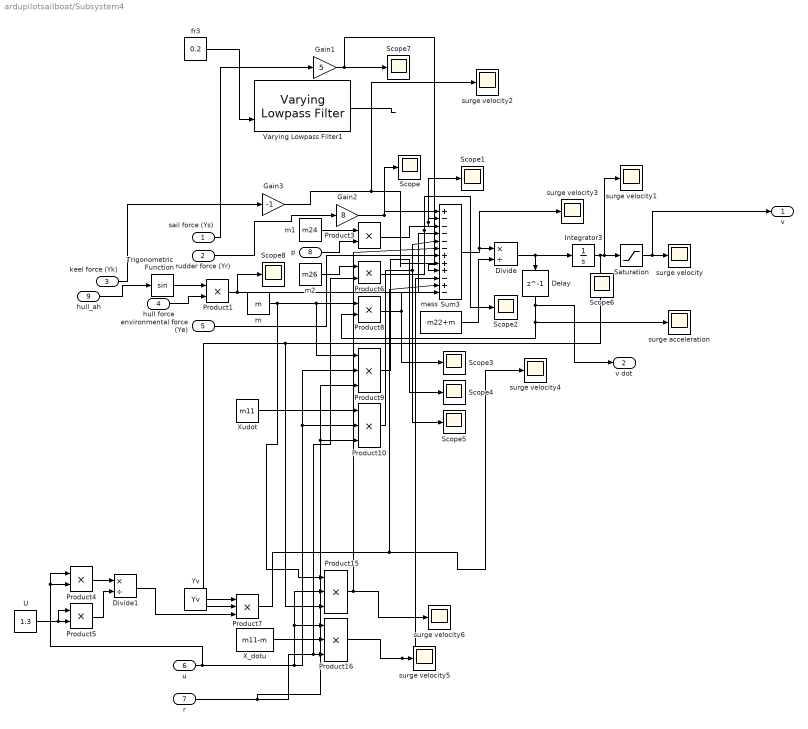
== system ardupilotsailboat/Subsystem4 ==
  sail force (Ys) : Inport
  rudder force (Yr) : Inport  Port=2
  keel force (Yk) : Inport  Port=3
  "hull force " : Inport  Port=4
  environmental force (Ye) : Inport  Port=5
  u : Inport  Port=6
  r : Inport  Port=7
  p : Inport  Port=8
  hull_ah : Inport  Port=9
  Delay : Delay  DelayLength=1  InitialCondition=0
  Divide : Product  Inputs=*/
  Divide1 : Product  Inputs=*/
  Gain1 : Gain  Gain=5
  Gain2 : Gain  Gain=8
  Gain3 : Gain  Gain=-1
  Integrator3 : Integrator  UpperSaturationLimit=0.01  LowerSaturationLimit=-0.01
  Product{1,3..6,8} (6 alike) : Product
  Product{7,9..10,15..16} (5 alike) : Product  Inputs=3
  Saturation : Saturate  UpperLimit=0.4  LowerLimit=-0.4
  Scope{,1..8} (9 alike) : Scope
  Sum3 : Sum  Inputs=|+-----+++-+-
  Trigonometric Function : Trigonometry
  U : Constant  Value=1.3
  Varying Lowpass Filter1 : cstblocks/Linear Parameter Varying/Varying Lowpass Filter  N=1
  X_dotu : Constant  Value=m11-m
  Xudot : Constant  Value=m11
  Yv : Constant  Value=Yv
  fr3 : Constant  Value=0.2
  m : Constant  Value=m
  m1 : Constant  Value=m24
  m2 : Constant  Value=m26
  mass : Constant  Value=m22+m
  surge acceleration : Scope
  surge velocity{,1..6} (7 alike) : Scope
  v : Outport
  v dot : Outport  Port=2
  wires:
  sail force (Ys)/1 -> Gain1/1
  mass/1 -> Divide/2
  Sum3/1 -> surge velocity3/1, Divide/1
  X_dotu/1 -> Product16/2
  Yv/1 -> Product7/1
  Product15/1 -> surge velocity6/1, Sum3/6
  Product16/1 -> surge velocity5/1, Sum3/10
  r/1 -> Product10/3, Product9/3, Product6/2, Product16/3
  fr3/1 -> Varying Lowpass Filter1/2
  Varying Lowpass Filter1/1 -> ?
  keel force (Yk)/1 -> Gain3/1
  Product5/1 -> Divide1/2
  U/1 -> Product5/1, Product5/2
  Product4/1 -> Divide1/1
  Divide1/1 -> Product7/3
  Integrator3/1 -> surge velocity1/1, Saturation/1, Product15/3, Product7/2
  m1/1 -> Product3/1
  Product3/1 -> Scope1/1, Sum3/2
  Product6/1 -> Scope2/1, Sum3/3
  m2/1 -> Product6/1
  Product8/1 -> Sum3/4, Scope3/1
  m/1 -> Product15/1, Product9/1, Product8/1
  u/1 -> Product10/2, Product9/2, Product16/1, Product15/2, Product4/1, Product4/2
  Xudot/1 -> Product10/1
  rudder force (Yr)/1 -> Gain2/1
  Product9/1 -> Scope4/1
  Product10/1 -> Sum3/5, Scope5/1
  Gain2/1 -> Scope/1, Sum3/1
  Gain1/1 -> Sum3/9, Scope7/1
  Gain3/1 -> Sum3/8, surge velocity2/1
  p/1 -> Product3/2
  Saturation/1 -> v/1, surge velocity/1
  environmental force (Ye)/1 -> Sum3/7
  Product7/1 -> Sum3/11, surge velocity4/1
  Divide/1 -> Delay/1, Integrator3/1
  Delay/1 -> v dot/1, Product8/2, surge acceleration/1
  "hull force "/1 -> Product1/2
  Product1/1 -> Scope8/1, Sum3/12
  Trigonometric Function/1 -> Product1/1
  hull_ah/1 -> Trigonometric Function/1

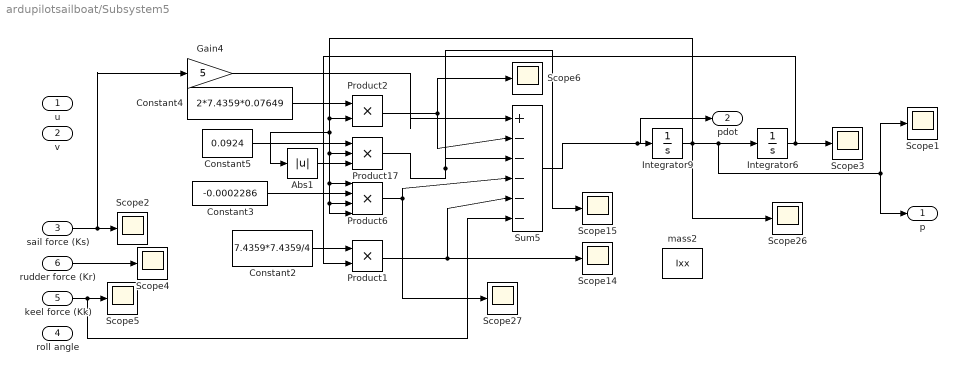
== system ardupilotsailboat/Subsystem5 ==
  u : Inport
  v : Inport  Port=2
  sail force (Ks) : Inport  Port=3
  roll angle : Inport  Port=4
  keel force (Kk) : Inport  Port=5
  rudder force (Kr) : Inport  Port=6
  Abs1 : Abs  SaturateOnIntegerOverflow=off
  Constant2 : Constant  Value=7.4359*7.4359/4
  Constant3 : Constant  Value=-0.0002286
  Constant4 : Constant  Value=2*7.4359*0.07649
  Constant5 : Constant  Value=0.0924
  Gain4 : Gain  Gain=5
  Integrator6 : Integrator
  Integrator9 : Integrator
  Product1 : Product
  Product17 : Product  Inputs=3
  Product2 : Product
  Product6 : Product  Inputs=4
  Scope{1..6,14..15,26..27} (10 alike) : Scope
  Sum5 : Sum  Inputs=|+-----
  mass2 : Constant  Value=Ixx
  p : Outport
  pdot : Outport  Port=2
  wires:
  Integrator9/1 -> Scope26/1, Product6/1, Product6/4, Product6/3, Product17/2, Abs1/1, Product2/2, Scope1/1, p/1, Integrator6/1
  Constant3/1 -> Product6/2
  Product2/1 -> Sum5/2, Scope6/1
  Sum5/1 -> pdot/1, Integrator9/1
  sail force (Ks)/1 -> Gain4/1, Scope2/1
  Constant4/1 -> Product2/1
  Abs1/1 -> Product17/3
  Constant5/1 -> Product17/1
  Constant2/1 -> Product1/1
  Product1/1 -> Sum5/5, Scope14/1
  Product6/1 -> Scope27/1, Sum5/4
  Product17/1 -> Scope15/1, Sum5/3
  Integrator6/1 -> Product1/2, Scope3/1
  rudder force (Kr)/1 -> Scope4/1
  keel force (Kk)/1 -> Sum5/6, Scope5/1
  Gain4/1 -> Sum5/1

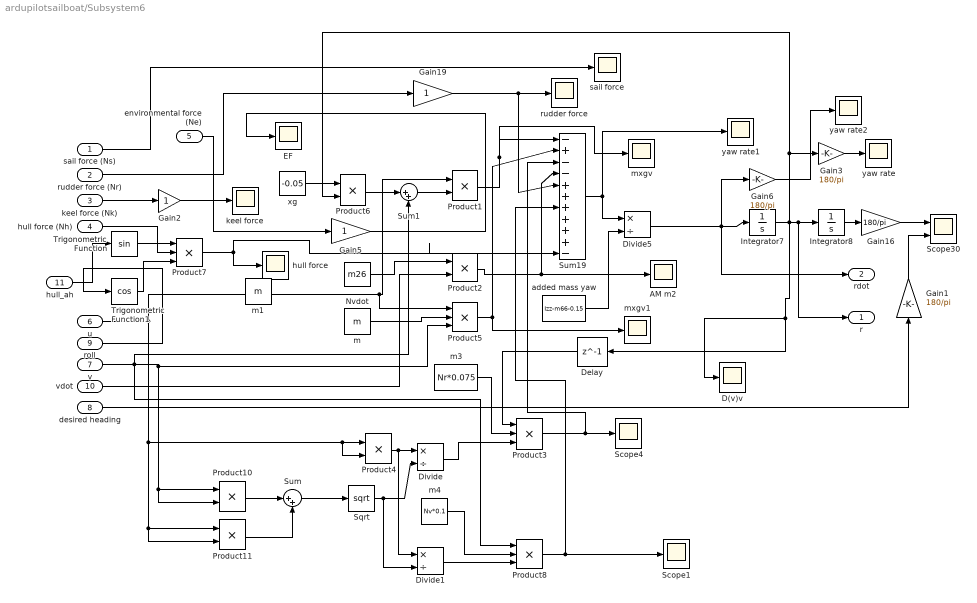
== system ardupilotsailboat/Subsystem6 ==
  sail force (Ns) : Inport
  rudder force (Nr) : Inport  Port=2
  keel force (Nk) : Inport  Port=3
  hull force (Nh) : Inport  Port=4
  environmental force (Ne) : Inport  Port=5
  u : Inport  Port=6
  v : Inport  Port=7
  desired heading : Inport  Port=8
  roll : Inport  Port=9
  vdot : Inport  Port=10
  hull_ah : Inport  Port=11
  AM m2 : Scope
  D(v)v : Scope
  Delay : Delay  DelayLength=1  InitialCondition=0
  Divide : Product  Inputs=*/
  Divide1 : Product  Inputs=*/
  Divide5 : Product  Inputs=*/
  EF : Scope
  Gain{1,3,6,16} (4 alike) : Gain  Gain=180/pi
  Gain19 : Gain
  Gain2 : Gain
  Gain5 : Gain
  Integrator7 : Integrator
  Integrator8 : Integrator
  Nvdot : Constant  Value=m26
  Product{1..2,4,6,10..11} (6 alike) : Product
  Product{3,5,7..8} (4 alike) : Product  Inputs=3
  Scope1 : Scope
  Scope30 : Scope  NumInputPorts=2
  Scope4 : Scope
  Sqrt : Sqrt
  Sum : Sum  Inputs=|++
  Sum1 : Sum  Inputs=|++
  Sum19 : Sum  Inputs=|-+--++++++-
  Trigonometric Function : Trigonometry
  Trigonometric Function1 : Trigonometry  Operator=cos
  added mass yaw : Constant  Value=Izz-m66-0.15  VectorParams1D=off
  hull force : Scope
  keel force : Scope
  m : Constant  Value=m
  m1 : Constant  Value=m
  m3 : Constant  Value=Nr*0.075
  m4 : Constant  Value=Nv*0.1
  mxgv : Scope
  mxgv1 : Scope
  rudder force : Scope
  sail force : Scope
  xg : Constant  Value=-0.05
  yaw rate : Scope
  yaw rate1 : Scope
  yaw rate2 : Scope
  r : Outport
  rdot : Outport  Port=2
  wires:
  Gain16/1 -> Scope30/1
  added mass yaw/1 -> Divide5/2
  Sum19/1 -> Divide5/1, yaw rate1/1
  sail force (Ns)/1 -> sail force/1
  rudder force (Nr)/1 -> Gain19/1
  environmental force (Ne)/1 -> Gain5/1
  u/1 -> Product1/1, Product5/1, Product11/2, Product11/1, Product4/2, Product4/1
  Nvdot/1 -> Product2/1
  desired heading/1 -> Gain1/1
  Integrator8/1 -> Gain16/1
  Gain1/1 -> Scope30/2
  Gain19/1 -> Sum19/5, rudder force/1
  keel force (Nk)/1 -> Gain2/1
  Gain2/1 -> keel force/1
  Integrator7/1 -> r/1, Integrator8/1, Delay/1, D(v)v/1, Product6/2, Gain3/1
  m3/1 -> Product3/2
  Product4/1 -> Divide/1, Divide1/1
  Sqrt/1 -> Divide1/2, Divide/2
  vdot/1 -> Product2/2
  Product8/1 -> Sum19/7, Scope1/1
  Product3/1 -> Sum19/3, Scope4/1
  m/1 -> Product5/2
  Product1/1 -> Sum19/1, mxgv/1
  Divide/1 -> Product3/3
  Product10/1 -> Sum/1
  Product11/1 -> Sum/2
  v/1 -> Product8/1, Product5/3, Product10/2, Product10/1, Sum1/2
  Sum/1 -> Sqrt/1
  m4/1 -> Product8/2
  Divide1/1 -> Product8/3
  Product2/1 -> Sum19/4, AM m2/1
  Product6/1 -> Sum1/1
  xg/1 -> Product6/1
  Sum1/1 -> Product1/2
  Product5/1 -> mxgv1/1, Sum19/2
  Gain5/1 -> EF/1
  Gain6/1 -> yaw rate2/1
  Delay/1 -> Product3/1
  Divide5/1 -> Gain6/1, Integrator7/1, rdot/1
  hull force (Nh)/1 -> Product7/2
  Trigonometric Function/1 -> Product7/1
  hull_ah/1 -> Trigonometric Function/1
  Product7/1 -> hull force/1, Sum19/11
  roll/1 -> Trigonometric Function1/1
  Trigonometric Function1/1 -> Product7/3
  Gain3/1 -> yaw rate/1

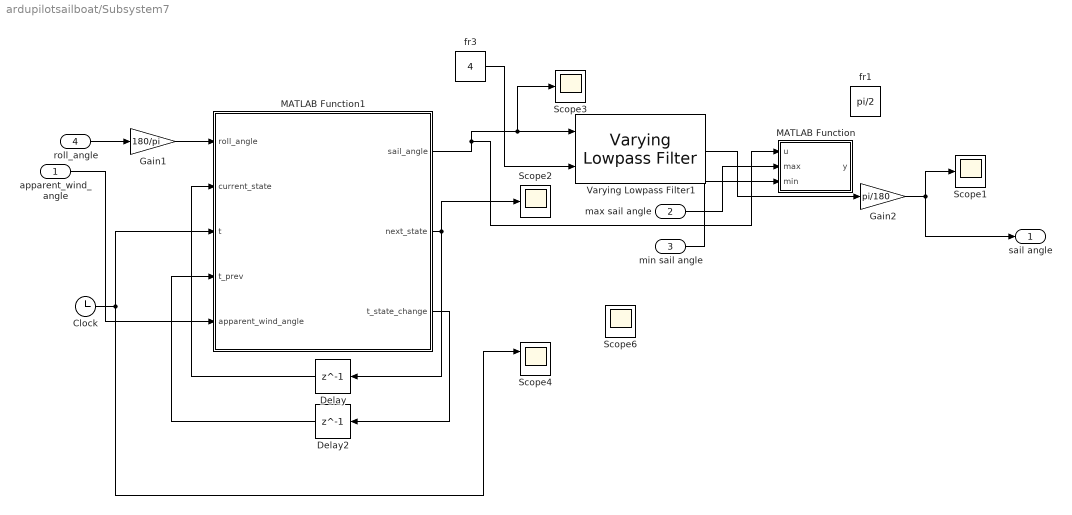
== system ardupilotsailboat/Subsystem7 ==
  apparent_wind_angle : Inport
  max sail angle : Inport  Port=2
  min sail angle : Inport  Port=3
  roll_angle : Inport  Port=4
  Clock : Clock
  Delay : Delay  DelayLength=1  InitialCondition=0
  Delay2 : Delay  DelayLength=1  InitialCondition=0
  Gain1 : Gain  Gain=180/pi
  Gain2 : Gain  Gain=pi/180
  MATLAB Function : MATLAB Function  TreatAsAtomicUnit=on
  MATLAB Function1 : MATLAB Function  TreatAsAtomicUnit=on
  Scope{1..3,6} (4 alike) : Scope
  Scope4 : Scope  NumInputPorts=2
  Varying Lowpass Filter1 : cstblocks/Linear Parameter Varying/Varying Lowpass Filter  N=1
  fr1 : Constant  Value=pi/2
  fr3 : Constant  Value=4
  sail angle : Outport
  wires:
  fr3/1 -> Varying Lowpass Filter1/2
  max sail angle/1 -> MATLAB Function/2(max)
  min sail angle/1 -> MATLAB Function/3(min)
  MATLAB Function1/2(next_state) -> Scope2/1, Delay/1
  MATLAB Function1/3(t_state_change) -> Delay2/1
  Clock/1 -> Scope4/1, MATLAB Function1/3(t)
  Varying Lowpass Filter1/1 -> Gain2/1
  Delay/1 -> MATLAB Function1/2(current_state)
  Delay2/1 -> MATLAB Function1/4(t_prev)
  MATLAB Function1/1(sail_angle) -> MATLAB Function/1(u), Varying Lowpass Filter1/1, Scope3/1
  apparent_wind_angle/1 -> MATLAB Function1/5(apparent_wind_angle)
  roll_angle/1 -> Gain1/1
  Gain1/1 -> MATLAB Function1/1(roll_angle)
  Gain2/1 -> Scope1/1, sail angle/1

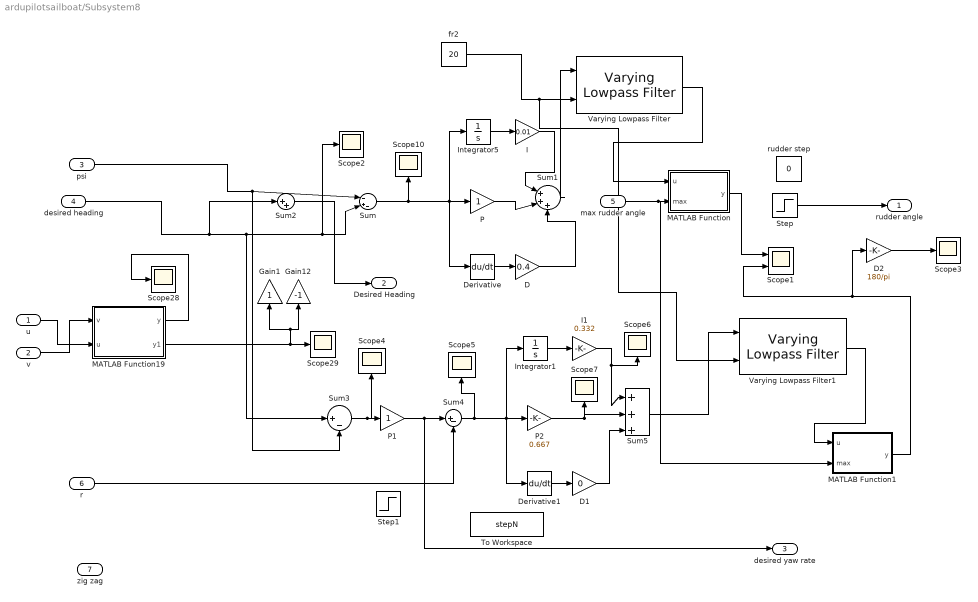
== system ardupilotsailboat/Subsystem8 ==
  u : Inport
  v : Inport  Port=2
  psi : Inport  Port=3
  desired heading : Inport  Port=4
  max rudder angle : Inport  Port=5
  r : Inport  Port=6
  zig zag : Inport  Port=7
  D : Gain  Gain=0.4
  D1 : Gain  Gain=0
  D2 : Gain  Gain=180/pi
  Derivative : Derivative
  Derivative1 : Derivative
  Gain1 : Gain
  Gain12 : Gain  Gain=-1
  I : Gain  Gain=0.01
  I1 : Gain  Gain=0.332
  Integrator1 : Integrator
  Integrator5 : Integrator
  MATLAB Function : MATLAB Function  TreatAsAtomicUnit=on
  MATLAB Function1 : MATLAB Function  TreatAsAtomicUnit=on
  MATLAB Function19 : MATLAB Function  TreatAsAtomicUnit=on
  P : Gain
  P1 : Gain
  P2 : Gain  Gain=0.667
  Scope1 : Scope  NumInputPorts=2
  Scope{2..7,10,28..29} (9 alike) : Scope
  Step : Step  Time=0.01  After=0.1945  SampleTime=0
  Step1 : Step  Time=5  After=0  SampleTime=0
  Sum : Sum  Inputs=|-+-
  Sum1 : Sum  Inputs=|+++
  Sum2 : Sum  Inputs=|++
  Sum3 : Sum  Inputs=|+-
  Sum4 : Sum  Inputs=|+-
  Sum5 : Sum  Inputs=|+++
  To Workspace : ToWorkspace  VariableName=stepN  SaveFormat=Timeseries  SampleTime=-1
  Varying Lowpass Filter : cstblocks/Linear Parameter Varying/Varying Lowpass Filter  N=1
  Varying Lowpass Filter1 : cstblocks/Linear Parameter Varying/Varying Lowpass Filter  N=1
  fr2 : Constant  Value=20
  rudder step : Constant  Value=0
  rudder angle : Outport
  Desired Heading : Outport  Port=2
  desired yaw rate : Outport  Port=3
  wires:
  Varying Lowpass Filter/1 -> MATLAB Function/1(u)
  MATLAB Function/1(y) -> Scope1/1
  Sum1/1 -> Varying Lowpass Filter/1
  I/1 -> Sum1/1
  Sum/1 -> Scope10/1, Derivative/1, Integrator5/1, P/1
  fr2/1 -> Varying Lowpass Filter/2, Varying Lowpass Filter1/2
  D/1 -> Sum1/3
  P/1 -> Sum1/2
  Derivative/1 -> D/1
  Integrator5/1 -> I/1
  MATLAB Function19/2(y1) -> Gain1/1, Gain12/1, Scope29/1
  MATLAB Function19/1(y) -> Scope28/1
  u/1 -> MATLAB Function19/2(u)
  v/1 -> MATLAB Function19/1(v)
  max rudder angle/1 -> MATLAB Function1/2(max), MATLAB Function/2(max)
  desired heading/1 -> Sum3/1, Sum/2, Scope2/1, Sum2/1
  Sum2/1 -> Desired Heading/1
  Sum3/1 -> Scope4/1, P1/1
  Sum4/1 -> Scope5/1, Derivative1/1, Integrator1/1, P2/1
  Integrator1/1 -> I1/1
  Derivative1/1 -> D1/1
  D1/1 -> Sum5/3
  Varying Lowpass Filter1/1 -> MATLAB Function1/1(u)
  psi/1 -> Sum3/2, Sum/1
  D2/1 -> Scope3/1
  P1/1 -> desired yaw rate/1, Sum4/1
  r/1 -> Sum4/2
  I1/1 -> Scope6/1, Sum5/1
  P2/1 -> Scope7/1, Sum5/2
  Sum5/1 -> Varying Lowpass Filter1/1
  MATLAB Function1/1(y) -> D2/1, Scope1/2
  Step/1 -> rudder angle/1

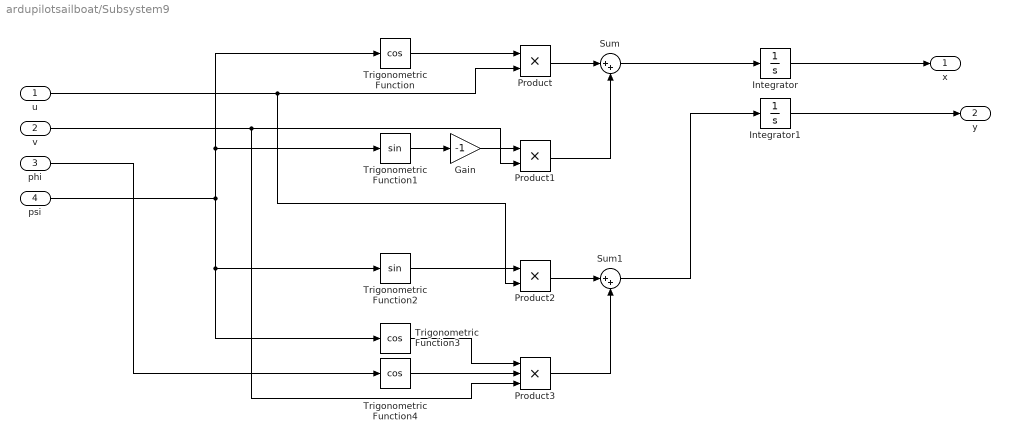
== system ardupilotsailboat/Subsystem9 ==
  u : Inport
  v : Inport  Port=2
  phi : Inport  Port=3
  psi : Inport  Port=4
  Gain : Gain  Gain=-1
  Integrator : Integrator
  Integrator1 : Integrator
  Product : Product
  Product1 : Product
  Product2 : Product
  Product3 : Product  Inputs=3
  Sum : Sum  Inputs=|++
  Sum1 : Sum  Inputs=|++
  Trigonometric Function : Trigonometry  Operator=cos
  Trigonometric Function1 : Trigonometry
  Trigonometric Function2 : Trigonometry
  Trigonometric Function3 : Trigonometry  Operator=cos
  Trigonometric Function4 : Trigonometry  Operator=cos
  x : Outport
  y : Outport  Port=2
  wires:
  Integrator/1 -> x/1
  Integrator1/1 -> y/1
  psi/1 -> Trigonometric Function1/1, Trigonometric Function/1, Trigonometric Function3/1, Trigonometric Function2/1
  Trigonometric Function/1 -> Product/1
  u/1 -> Product/2, Product2/2
  Trigonometric Function1/1 -> Gain/1
  Gain/1 -> Product1/1
  v/1 -> Product1/2, Product3/3
  Product/1 -> Sum/1
  Product1/1 -> Sum/2
  Sum/1 -> Integrator/1
  Product3/1 -> Sum1/2
  Sum1/1 -> Integrator1/1
  Trigonometric Function2/1 -> Product2/1
  Product2/1 -> Sum1/1
  Trigonometric Function3/1 -> Product3/1
  Trigonometric Function4/1 -> Product3/2
  phi/1 -> Trigonometric Function4/1
